simulink model "H_g_Greska_inverzna_staticka_karakteristika_Nepotpuna_tabela"  (R2016a)
settings: Solver=VariableStepAuto  StartTime=0.0  StopTime=800  RelTol=1e-3
libraries: simulink x2
settings Model: Creator=AmelT  LastModifiedBy=AmelT

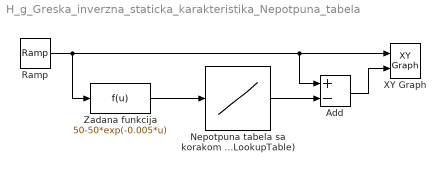
== system H_g_Greska_inverzna_staticka_karakteristika_Nepotpuna_tabela ==
  Add : Sum  Inputs=+-
  Nepotpuna tabela sa korakom 100 (0,800)   (1-D LookupTable) : Lookup_n-D  NumberOfTableDimensions=1  BreakpointsForDimension1=50-50*exp(-0.005*[0:100:800])  Table=[0:100:800]  InternalRulePriority=Speed  RndMeth=Simplest  InputSameDT=on
  Ramp : simulink/Sources/Ramp  slope=1  start=0  X0=0
  XY Graph : simulink/Sinks/XY Graph  xmin=0  xmax=800  ymin=-10  ymax=10  st=1
  Zadana funkcija : Fcn  Expr=50-50*exp(-0.005*u)
  wires:
  Zadana funkcija/1 -> Nepotpuna tabela sa korakom 100 (0,800)   (1-D LookupTable)/1
  Ramp/1 -> Zadana funkcija/1, Add/1, XY Graph/1
  Nepotpuna tabela sa korakom 100 (0,800)   (1-D LookupTable)/1 -> Add/2
  Add/1 -> XY Graph/2
